simulink model "evenorder_twolevel"  (R2015b)
settings: Solver=VariableStepAuto  StartTime=0.0  StopTime=0.5  RelTol=1e-3
libraries: powerlib x13, simulink x3
settings Model: Creator=hakan  LastModifiedBy=hakan

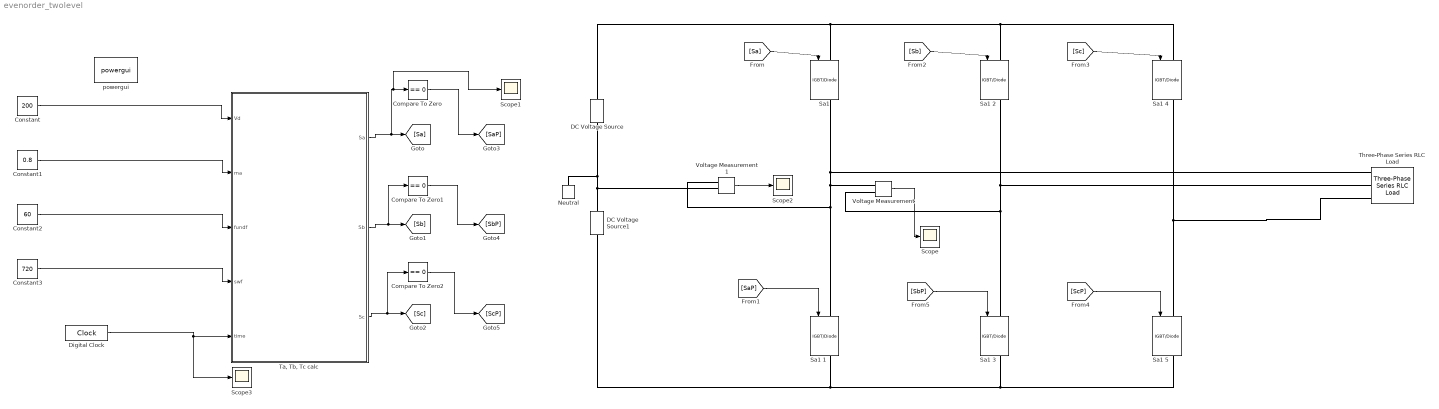
== system evenorder_twolevel ==
  Compare To Zero : simulink/Logic and Bit Operations/Compare To Zero  relop===  OutDataTypeStr=boolean
  Compare To Zero1 : simulink/Logic and Bit Operations/Compare To Zero  relop===  OutDataTypeStr=boolean
  Compare To Zero2 : simulink/Logic and Bit Operations/Compare To Zero  relop===  OutDataTypeStr=boolean
  Constant : Constant  Value=200
  Constant1 : Constant  Value=0.8
  Constant2 : Constant  Value=60
  Constant3 : Constant  Value=720  VectorParams1D=off
  DC Voltage Source : powerlib/Electrical Sources/DC Voltage Source  Amplitude=100  Measurements=Voltage
  DC Voltage Source1 : powerlib/Electrical Sources/DC Voltage Source  Amplitude=100  Measurements=Voltage
  Digital Clock : DigitalClock  SampleTime=0.0000001
  Neutral : powerlib/Elements/Neutral  LConnTagsString=a  NodeNumber=10
  Sa1 {,1..5} (6 alike) : powerlib/Power Electronics/IGBT//Diode  Ron=1e-3  Rs=1e5  Cs=inf  Measurements=on
  Scope{,1..3} (4 alike) : Scope
  "Ta, Tb, Tc calc" : MATLAB Function  TreatAsAtomicUnit=on
  Three-Phase Series RLC Load : powerlib/Elements/Three-Phase Series RLC Load  LConnTagsString=A|B|C  Configuration=Y (grounded)  NominalVoltage=1000  Vabc=[1e3 1e3 1e3]  Vabcp=[1e3 1e3 1e3]  NominalFrequency=50  UnbalancedPower=off  ActivePower=10000  InductivePower=4000  CapacitivePower=0  Pabc=[10e3 9e3 11e3]  QLabc=[100 90 110]  QCabc=[100 90 110]  Pabcp=[10e3 9e3 11e3]  QLabcp=[100 90 110]  QCabcp=[100 90 110]  Measurements=None  LoadType=constant Z
  Voltage Measurement : powerlib/Measurements/Voltage Measurement  PhasorSimulation=off  OutputType=Complex  PSBequivalent=0
  Voltage Measurement1 : powerlib/Measurements/Voltage Measurement  PhasorSimulation=off  OutputType=Complex  PSBequivalent=0
  powergui : powerlib/powergui  Priority=1  SimulationMode=Continuous  SolverType=Tustin/Backward Euler (TBE)  SampleTime=50e-6  frequency=60  SPID=off  DisableSnubberDevices=off  DisableRonSwitches=off  DisableVfSwitches=off  SwTol=0  DisplayEquations=off  Interpol=off  ExternalGateDelay=off  methode=off  Ts=10  FunctionMessages=off  echomessages=off  HookPort=off  EnableUseOfTLC=off  x0status=blocks  frequencyindice=0  Pbase=100e6  ErrMax=1e-4  Iterations=50  UnitsV=kV  UnitsW=MW  buscounter=0  RestoreLinks=warning  ResistiveCurrentMeasurement=off  Frange=[0:2:500]  Ylog=off  Xlog=on  ShowGrid=off  save=off  variable=ZData  structure=linetoline  ZoomFFT=off  StartTime=0.0  cycles=2  DisplayStyle=1  fundamental=50  FreqAxis=off  MaxFrequency=5000  frequencyindicesteady=1  RmsSteady=1  display=off
  wires:
  "Ta, Tb, Tc calc"/1(Sa) -> Scope1/1, Compare To Zero/1, [Sa]
  "Ta, Tb, Tc calc"/2(Sb) -> Compare To Zero1/1, [Sb]
  "Ta, Tb, Tc calc"/3(Sc) -> Compare To Zero2/1, [Sc]
  Compare To Zero/1 -> [SaP]
  Compare To Zero1/1 -> [SbP]
  Compare To Zero2/1 -> [ScP]
  [Sa] -> "Sa1 "/1
  [SaP] -> Sa1 1/1
  [Sb] -> Sa1 2/1
  [SbP] -> Sa1 3/1
  [Sc] -> Sa1 4/1
  [ScP] -> Sa1 5/1
  Voltage Measurement/1 -> Scope/1
  Constant/1 -> "Ta, Tb, Tc calc"/1(Vd)
  Constant1/1 -> "Ta, Tb, Tc calc"/2(ma)
  Constant2/1 -> "Ta, Tb, Tc calc"/3(fundf)
  Constant3/1 -> "Ta, Tb, Tc calc"/4(swf)
  Digital Clock/1 -> Scope3/1, "Ta, Tb, Tc calc"/5(time)
  Voltage Measurement1/1 -> Scope2/1
  connections:
  "Sa1 "/LConn1 -- DC Voltage Source/RConn1 -- Sa1 4/LConn1 -- Sa1 2/LConn1
  Voltage Measurement/LConn1 -- Voltage Measurement1/LConn1 -- Sa1 1/LConn1 -- "Sa1 "/RConn1 -- Three-Phase Series RLC Load/LConn1
  Sa1 3/LConn1 -- Voltage Measurement/LConn2 -- Sa1 2/RConn1 -- Three-Phase Series RLC Load/LConn2
  Sa1 5/LConn1 -- Sa1 4/RConn1 -- Three-Phase Series RLC Load/LConn3
  Sa1 1/RConn1 -- DC Voltage Source1/LConn1 -- Sa1 3/RConn1 -- Sa1 5/RConn1
  Neutral/LConn1 -- Voltage Measurement1/LConn2 -- DC Voltage Source1/RConn1 -- DC Voltage Source/LConn1

== matlab function evenorder_twolevel/Ta, Tb, Tc calc ==
  data: Sa output; Sb output; Vd input; ma input; fundf input; swf input; time input; Sc output
function [Sa, Sb, Sc] = fcn(Vd,ma,fundf, swf, time)
% this program works for magnitude of Vref is greater then Vd/3 meaning ma
% must be greater than 1/sqrt(3). for smaller ma's computation is a bit
% more tricky therefore it is omitted for simplicity for now. 
Vref = ma*Vd/sqrt(3); %magnitude of Vref
theta = 2*pi*fundf*time; %angle of Vref
angle = mod(theta, 2*pi);
Ts = 1/swf;
Ta = 0;
Tb = 0;
Tc = 0;
T0 = 0;
n=0;
output = 0;
%Sector1 = 0; Sector2 = 0; Sector3 = 0; Sector4= 0; Sector5 = 0; Sector6 = 0;
Sa=0; Sb=0; Sc=0;
timee = mod(time,Ts);
        va= [0 0 0 0 0 0 0];
        vb= [0 0 0 0 0 0 0];
        vc= [0 0 0 0 0 0 0];


%% Sector 1
if (mod(theta, 2*pi)<=pi/3)&&(mod(theta, 2*pi)>0)  % sector 1
    n = 1;
    thetaprime = angle - (n-1)*pi/3;
    
    Ta = Ts*ma*sin(pi/3-thetaprime);
    Tb = Ts*ma*sin(thetaprime);
    T0 = Ts-Ta-Tb;
    
    
    
    times = [T0/4 Ta/2 Tb/2 T0/2 Tb/2 Ta/2 T0/4];
    times = cumsum(times);
    if (angle>0)&&(angle<=pi/6)  % then 1a
        va= [0 1 1 1 1 1 0];
        vb= [0 0 1 1 1 0 0];
        vc= [0 0 0 1 0 0 0];
    end
    
    if (angle>pi/6)&&(angle<=pi/3)  % then 1b
        va= [1 1 1 0 1 1 1];
        vb= [1 1 0 0 0 1 1];
        vc= [1 0 0 0 0 0 1];
    end
    
    
    
    for j = 1:7            
            if(timee<times(j))
                break
            end
    end
        Sa=va(j); 
        Sb=vb(j); 
        Sc=vc(j); 
end
%% Sector 2
if (mod(theta, 2*pi)<=2*pi/3)&&(mod(theta, 2*pi)>pi/3)  % sector 2
    n = 2;
    thetaprime = angle - (n-1)*pi/3;
    
    Ta = Ts*ma*sin(pi/3-thetaprime);
    Tb = Ts*ma*sin(thetaprime);
    T0 = Ts-Ta-Tb;   
    
    times = [T0/4 Ta/2 Tb/2 T0/2 Tb/2 Ta/2 T0/4];
    times = cumsum(times);

    if (angle>pi/3)&&(angle<=pi/2)  % then 2a
        va= [1 1 0 0 0 1 1];
        vb= [1 1 1 0 1 1 1];
        vc= [1 0 0 0 0 0 1];
    end
    
    if (angle>pi/2)&&(angle<=2*pi/3)  % then 2b
        va= [0 0 1 1 1 0 0];
        vb= [0 1 1 1 1 1 0];
        vc= [0 0 0 1 0 0 0];
    end
        
    
    for j = 1:7            
            if(timee<times(j))
                break
            end
    end
        Sa=va(j); 
        Sb=vb(j); 
        Sc=vc(j); 
end


%% Sector 3
if (mod(theta, 2*pi)<=pi)&&(mod(theta, 2*pi)>2*pi/3)  % sector 3
    n = 3;
    thetaprime = angle - (n-1)*pi/3;
    
    Ta = Ts*ma*sin(pi/3-thetaprime);
    Tb = Ts*ma*sin(thetaprime);
    T0 = Ts-Ta-Tb;  
    
    times = [T0/4 Ta/2 Tb/2 T0/2 Tb/2 Ta/2 T0/4];
    times = cumsum(times);
    
    if (angle>2*pi/3)&&(angle<=5*pi/6)  % then 3a
        va= [0 0 0 1 0 0 0];
        vb= [0 1 1 1 1 1 0];
        vc= [0 0 1 1 1 0 0];
    end
    
    if (angle>5*pi/6)&&(angle<=pi)  % then 3b
        va= [1 0 0 0 0 0 1];
        vb= [1 1 1 0 1 1 1];
        vc= [1 1 0 0 0 1 1];
    end
    for j = 1:7            
            if(timee<times(j))
                break
            end
    end
        Sa=va(j); 
        Sb=vb(j); 
        Sc=vc(j);     
end


%% Sector 4
if (mod(theta, 2*pi)<=4*pi/3)&&(mod(theta, 2*pi)>pi)  % sector 4
    n = 4;
    thetaprime = angle - (n-1)*pi/3;
    
    Ta = Ts*ma*sin(pi/3-thetaprime);
    Tb = Ts*ma*sin(thetaprime);
    T0 = Ts-Ta-Tb;
    
    times = [T0/4 Ta/2 Tb/2 T0/2 Tb/2 Ta/2 T0/4];
    times = cumsum(times);
    
    if (angle>pi)&&(angle<=7*pi/6)  % then 4a
        va= [1 0 0 0 0 0 1];
        vb= [1 1 0 0 0 1 1];
        vc= [1 1 1 0 1 1 1];
    end
    
    if (angle>7*pi/6)&&(angle<=4*pi/3)  % then 4b
        va= [0 0 0 1 0 0 0];
        vb= [0 0 1 1 1 0 0];
        vc= [0 1 1 1 1 1 0];
    end
    
    
    for j = 1:7            
            if(timee<times(j))
                break
            end
    end
        Sa=va(j); 
        Sb=vb(j); 
        Sc=vc(j); 
    
end


%% Sector 5 
if (mod(theta, 2*pi)<=5*pi/3)&&(mod(theta, 2*pi)>4*pi/3)  % sector 5
    n = 5;
    thetaprime = angle - (n-1)*pi/3;
    
    Ta = Ts*ma*sin(pi/3-thetaprime);
    Tb = Ts*ma*sin(thetaprime);
    T0 = Ts-Ta-Tb;
    
    times = [T0/4 Ta/2 Tb/2 T0/2 Tb/2 Ta/2 T0/4];
    times = cumsum(times);
    
    if (angle>4*pi/3)&&(angle<=3*pi/2)  % then 5a
        va= [0 0 1 1 1 0 0];
        vb= [0 0 0 1 0 0 0];
        vc= [0 1 1 1 1 1 0];
    end
    
    if (angle>3*pi/2)&&(angle<=5*pi/3)  % then 5b
        va= [1 1 0 0 0 1 1];
        vb= [1 0 0 0 0 0 1];
        vc= [1 1 1 0 1 1 1];
    end
    
    for j = 1:7            
            if(timee<times(j))
                break
            end
    end
        Sa=va(j); 
        Sb=vb(j); 
        Sc=vc(j); 
    
end


%% Sector 6 
if (mod(theta, 2*pi)<=2*pi)&&(mod(theta, 2*pi)>5*pi/3)  % sector 6
    n = 6;
    thetaprime = angle - (n-1)*pi/3;
    
    Ta = Ts*ma*sin(pi/3-thetaprime);
    Tb = Ts*ma*sin(thetaprime);
    T0 = Ts-Ta-Tb;
    
    times = [T0/4 Ta/2 Tb/2 T0/2 Tb/2 Ta/2 T0/4];
    times = cumsum(times);
    
    if (angle>5*pi/3)&&(angle<=11*pi/6)  % then 6a
        va= [1 1 1 0 1 1 1];
        vb= [1 0 0 0 0 0 1];
        vc= [1 1 0 0 0 1 1];
    end
    
    if (angle>11*pi/6)&&(angle<=2*pi)  % then 6b
        va= [0 1 1 1 1 1 0];
        vb= [0 0 0 1 0 0 0];
        vc= [0 0 1 1 1 0 0];
    end
    
    for j = 1:7            
            if(timee<times(j))
                break
            end
    end
        Sa=va(j); 
        Sb=vb(j); 
        Sc=vc(j); 
end
